simulink model "Block_Diagram_Variables"  (R2024b)
settings: Solver=VariableStepAuto  StartTime=0.0  StopTime=10.0  RelTol=1e-3
undefined symbols (not defined in the file): R1, RV1, RV2
settings Model: Creator=Snoozer  LastModifiedBy=Snoozer

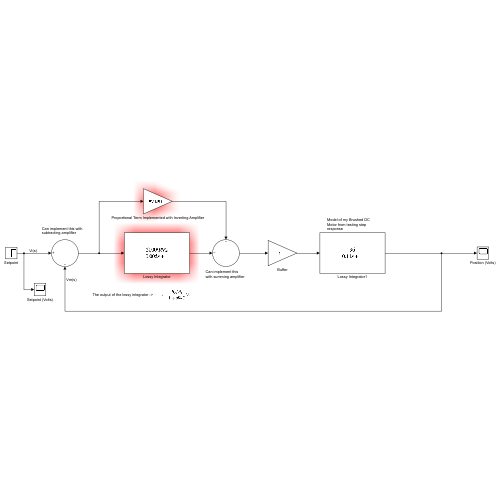
[thumbnail: Simulink's stored preview of the top-level diagram]
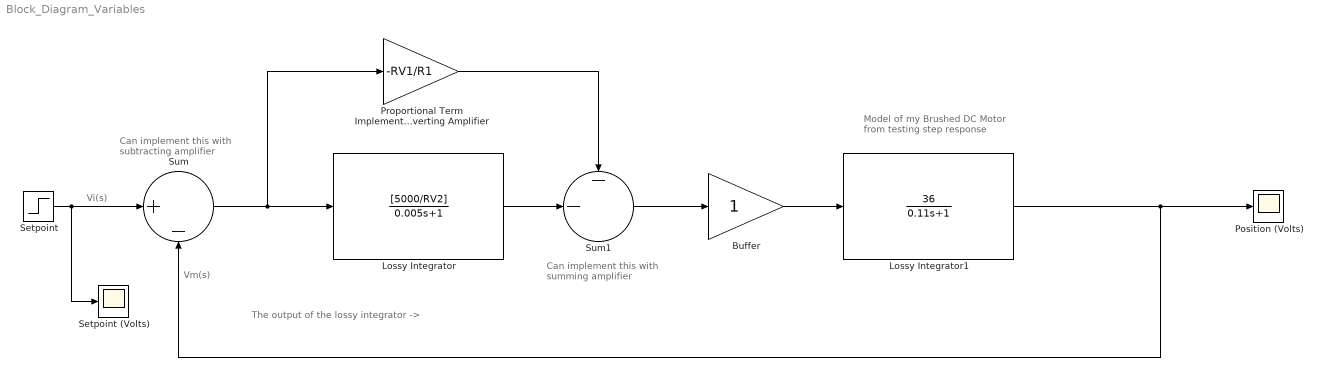
== system Block_Diagram_Variables ==
  note: Model of my Brushed DC Motor from testing step response
  note: Can implement this with subtracting amplifier
  note: Vi(s)
  note: Can implement this with summing amplifier
  note: The output of the lossy integrator ->
  note: Vm(s)
  Buffer : Gain
  Lossy Integrator : TransferFcn  Numerator=[5000/RV2]  Denominator=[0.005 1]
  Lossy Integrator1 : TransferFcn  Numerator=36  Denominator=[0.11 1]
  Position (Volts) : Scope
  Proportional Term Implemented with Inverting Amplifier : Gain  Gain=-RV1/R1
  Setpoint : Step  After=3  SampleTime=0
  Setpoint (Volts) : Scope
  Sum : Sum  Inputs=|+-
  Sum1 : Sum  Inputs=--|
  wires:
  Lossy Integrator/1 -> Sum1/2
  Setpoint/1 -> Setpoint (Volts)/1, Sum/1
  Sum/1 -> Proportional Term Implemented with Inverting Amplifier/1, Lossy Integrator/1
  Sum1/1 -> Buffer/1
  Buffer/1 -> Lossy Integrator1/1
  Proportional Term Implemented with Inverting Amplifier/1 -> Sum1/1
  Lossy Integrator1/1 -> Position (Volts)/1, Sum/2
